simulink model "pidparallel"  (R2022b)
settings: Solver=VariableStepAuto  StartTime=0.0  StopTime=.8  RelTol=1e-3
undefined symbols (not defined in the file): DiscIntNeverNeededParam
libraries: spsSeriesRLCBranchLib x7, spsCurrentMeasurementLib x4, spsDCVoltageSourceLib x2, spsDiodeLib x2, spsMosfetLib x2, spsSawtoothGeneratorLib x2, spsVoltageMeasurementLib x2, sps_lib x1
settings Model: Creator=User  LastModifiedBy=User

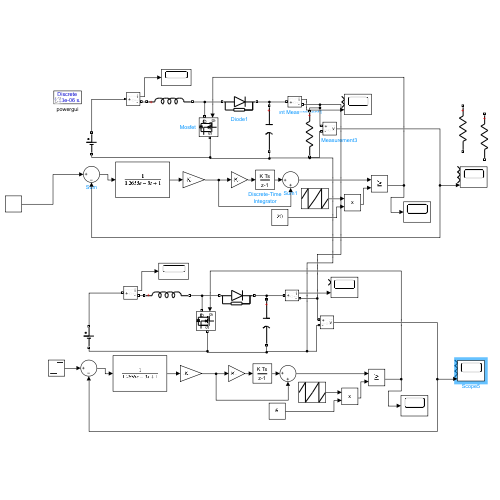
[thumbnail: Simulink's stored preview of the top-level diagram]
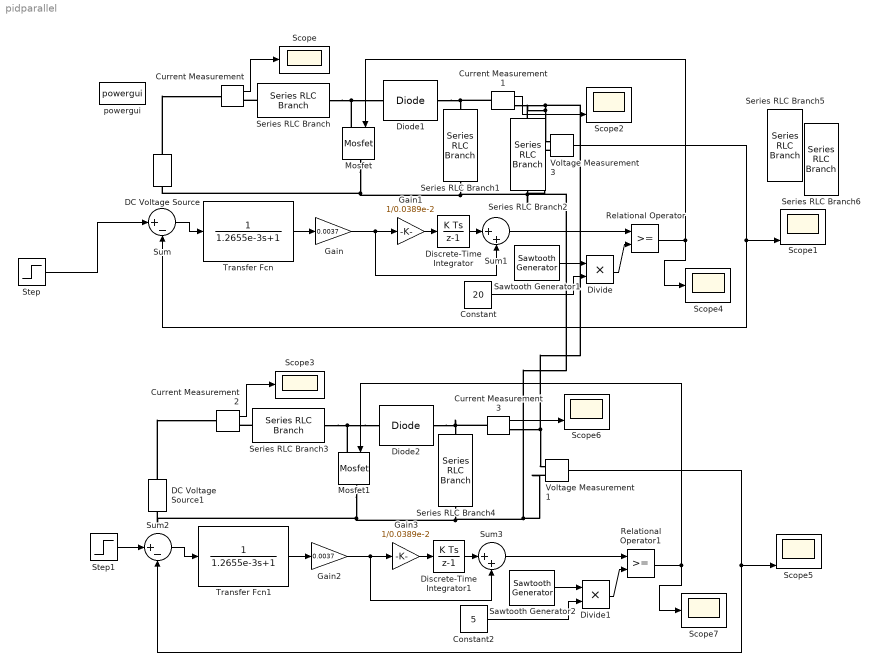
== system pidparallel ==
  Constant : Constant  Value=20
  Constant2 : Constant  Value=5
  Current Measurement{,1..3} (4 alike) : spsCurrentMeasurementLib/Current Measurement  PhasorSimulation=off  OutputType=Complex  PSBequivalent=0
  DC Voltage Source : spsDCVoltageSourceLib/DC Voltage Source  Amplitude=5  Measurements=None
  DC Voltage Source1 : spsDCVoltageSourceLib/DC Voltage Source  Amplitude=15  Measurements=None
  Diode1 : spsDiodeLib/Diode  Ron=0.001  Lon=0  Vf=0.8  IC=0  UseSnubber=0  Rs=500  Cs=250e-9  Measurements=off
  Diode2 : spsDiodeLib/Diode  Ron=0.001  Lon=0  Vf=0.8  IC=0  UseSnubber=0  Rs=500  Cs=250e-9  Measurements=off
  Discrete-Time Integrator : DiscreteIntegrator  SampleTime=1.33e-6  ICPrevOutput=DiscIntNeverNeededParam  ICPrevScaledInput=DiscIntNeverNeededParam
  Discrete-Time Integrator1 : DiscreteIntegrator  SampleTime=1.33e-6  ICPrevOutput=DiscIntNeverNeededParam  ICPrevScaledInput=DiscIntNeverNeededParam
  Divide : Product  Inputs=**
  Divide1 : Product  Inputs=**
  Gain : Gain  Gain=0.0037
  Gain1 : Gain  Gain=1/0.0389e-2
  Gain2 : Gain  Gain=0.0037
  Gain3 : Gain  Gain=1/0.0389e-2
  Mosfet : spsMosfetLib/Mosfet  Ron=0.1  Lon=0  Rd=0.01  Vfd=0  IC=0  Rs=1e5  Cs=inf  Measurements=off
  Mosfet1 : spsMosfetLib/Mosfet  Ron=0.1  Lon=0  Rd=0.01  Vfd=0  IC=0  Rs=1e5  Cs=inf  Measurements=off
  Relational Operator : RelationalOperator  OutDataTypeStr=boolean  RndMeth=Simplest  InputSameDT=off
  Relational Operator1 : RelationalOperator  OutDataTypeStr=boolean  RndMeth=Simplest  InputSameDT=off
  Sawtooth Generator1 : spsSawtoothGeneratorLib/Sawtooth Generator  Freq=15e3  Phase=180  Ts=1.33e-6
  Sawtooth Generator2 : spsSawtoothGeneratorLib/Sawtooth Generator  Freq=15e3  Phase=180  Ts=1.33e-6
  Scope{,3..4,7} (4 alike) : Scope
  Scope1 : Scope  NumInputPorts=4
  Scope2 : Scope  NumInputPorts=3
  Scope5 : Scope  NumInputPorts=4
  Scope6 : Scope  NumInputPorts=2
  Series RLC Branch : spsSeriesRLCBranchLib/Series RLC Branch  LConnTagsString=__new0  RConnTagsString=__new0  BranchType=L  Resistance=0  Inductance=1e-3  SetiL0=off  InitialCurrent=0  Capacitance=inf  Setx0=off  InitialVoltage=0  Measurements=None
  Series RLC Branch1 : spsSeriesRLCBranchLib/Series RLC Branch  LConnTagsString=__new0  RConnTagsString=__new0  BranchType=C  Resistance=0  Inductance=115.2e-6  SetiL0=off  InitialCurrent=0  Capacitance=330e-6  Setx0=off  InitialVoltage=0  Measurements=None
  Series RLC Branch2 : spsSeriesRLCBranchLib/Series RLC Branch  LConnTagsString=__new0  RConnTagsString=__new0  BranchType=R  Resistance=30  Inductance=115.2e-6  SetiL0=off  InitialCurrent=0  Capacitance=inf  Setx0=off  InitialVoltage=0  Measurements=None
  Series RLC Branch3 : spsSeriesRLCBranchLib/Series RLC Branch  LConnTagsString=__new0  RConnTagsString=__new0  BranchType=L  Resistance=0  Inductance=1e-3  SetiL0=off  InitialCurrent=0  Capacitance=inf  Setx0=off  InitialVoltage=0  Measurements=None
  Series RLC Branch4 : spsSeriesRLCBranchLib/Series RLC Branch  LConnTagsString=__new0  RConnTagsString=__new0  BranchType=C  Resistance=0  Inductance=115.2e-6  SetiL0=off  InitialCurrent=0  Capacitance=330e-6  Setx0=off  InitialVoltage=0  Measurements=None
  Series RLC Branch5 : spsSeriesRLCBranchLib/Series RLC Branch  LConnTagsString=__new0  RConnTagsString=__new0  BranchType=R  Resistance=30  Inductance=115.2e-6  SetiL0=off  InitialCurrent=0  Capacitance=inf  Setx0=off  InitialVoltage=0  Measurements=None
  Series RLC Branch6 : spsSeriesRLCBranchLib/Series RLC Branch  LConnTagsString=__new0  RConnTagsString=__new0  BranchType=R  Resistance=30  Inductance=115.2e-6  SetiL0=off  InitialCurrent=0  Capacitance=inf  Setx0=off  InitialVoltage=0  Measurements=None
  Step : Step  Time=0.4  Before=10  After=30  SampleTime=0
  Step1 : Step  Time=.2  After=10  SampleTime=0
  Sum : Sum  Inputs=|+-
  Sum1 : Sum  Inputs=|++
  Sum2 : Sum  Inputs=|+-
  Sum3 : Sum  Inputs=|++
  Transfer Fcn : TransferFcn  Denominator=[1.2655e-3 1]
  Transfer Fcn1 : TransferFcn  Denominator=[1.2655e-3 1]
  Voltage Measurement1 : spsVoltageMeasurementLib/Voltage Measurement  PhasorSimulation=off  OutputType=Complex  PSBequivalent=0
  Voltage Measurement3 : spsVoltageMeasurementLib/Voltage Measurement  PhasorSimulation=off  OutputType=Complex  PSBequivalent=0
  powergui : sps_lib/powergui  Priority=1  SimulationMode=Discrete  SampleTime=1.33e-6  frequency=60  Iterations=50  frequencyindice=0  Pbase=100e6  ErrMax=1e-4  UnitsV=kV  UnitsW=MW  buscounter=0  FunctionMessages=off  echomessages=off  EnableUseOfTLC=off  CurrentSourceSwitches=off  DisableSnubberDevices=off  DisableRonSwitches=off  DisableVfSwitches=off  DisplayEquations=off  AutomaticDiscreteSolvers=off  SolverType=Tustin/Backward Euler (TBE)  Interpol=off  ExternalGateDelay=off  methode=off  Ts=100  x0status=blocks  SPID=on  SwTol=0  HookPort=off  NonlinearTolerance=1e-4  nMaxIteration=100  ContinueOnMaxIteration=off  RestoreLinks=warning  ResistiveCurrentMeasurement=off  Frange=[0:2:500]  Ylog=off  Xlog=on  ShowGrid=off  save=off  variable=ZData  structure=0  ZoomFFT=off  StartTime=0.0  cycles=1  DisplayStyle=1  fundamental=60  FreqAxis=off  MaxFrequency=1000  frequencyindicesteady=1  RmsSteady=1  display=off
  wires:
  Divide/1 -> Relational Operator/2
  Sawtooth Generator1/1 -> Divide/1
  Constant/1 -> Divide/2
  Transfer Fcn/1 -> Gain/1
  Sum/1 -> Transfer Fcn/1
  Voltage Measurement3/1 -> Sum/2, Scope1/4
  Current Measurement/1 -> Scope/1
  Gain/1 -> Gain1/1, Sum1/2
  Discrete-Time Integrator/1 -> Sum1/1
  Sum1/1 -> Relational Operator/1
  Step/1 -> Sum/1
  Current Measurement1/1 -> Scope2/3
  Gain1/1 -> Discrete-Time Integrator/1
  Relational Operator/1 -> Scope4/1, Mosfet/1
  Discrete-Time Integrator1/1 -> Sum3/1
  Current Measurement3/1 -> Scope6/2
  Gain2/1 -> Gain3/1, Sum3/2
  Sum2/1 -> Transfer Fcn1/1
  Step1/1 -> Sum2/1
  Current Measurement2/1 -> Scope3/1
  Voltage Measurement1/1 -> Sum2/2, Scope5/4
  Constant2/1 -> Divide1/2
  Divide1/1 -> Relational Operator1/2
  Sawtooth Generator2/1 -> Divide1/1
  Sum3/1 -> Relational Operator1/1
  Relational Operator1/1 -> Scope7/1, Mosfet1/1
  Transfer Fcn1/1 -> Gain2/1
  Gain3/1 -> Discrete-Time Integrator1/1
  connections:
  Current Measurement3/RConn1 -- Voltage Measurement1/LConn1 -- Current Measurement1/RConn1 -- Series RLC Branch2/LConn1 -- Voltage Measurement3/LConn1
  DC Voltage Source1/LConn1 -- Voltage Measurement1/LConn2 -- Series RLC Branch1/RConn1 -- Mosfet/RConn1 -- DC Voltage Source/LConn1 -- Series RLC Branch2/RConn1 -- Voltage Measurement3/LConn2 -- Series RLC Branch4/RConn1 -- Mosfet1/RConn1
  Series RLC Branch/RConn1 -- Mosfet/LConn1 -- Diode1/LConn1
  Current Measurement1/LConn1 -- Diode1/RConn1 -- Series RLC Branch1/LConn1
  DC Voltage Source/RConn1 -- Current Measurement/LConn1
  Series RLC Branch/LConn1 -- Current Measurement/RConn1
  Diode2/LConn1 -- Series RLC Branch3/RConn1 -- Mosfet1/LConn1
  Series RLC Branch4/LConn1 -- Current Measurement3/LConn1 -- Diode2/RConn1
  DC Voltage Source1/RConn1 -- Current Measurement2/LConn1
  Series RLC Branch3/LConn1 -- Current Measurement2/RConn1
